simulink model "yangguo_Hermite_ISCAS2014_v03Final"  (Simulink 8.0)
settings: Solver=ode45  StartTime=0  StopTime=2e-8  FixedStep=Auto  MaxStep=1e-11  RelTol=1e-3
undefined symbols (not defined in the file or in its folder): tau
libraries: simulink x1
settings Model: Creator=yangguo  LastModifiedBy=Kushal
settings DataIOCC: SignalLoggingSaveFormat=ModelDataLogs
settings DebuggingCC: FcnCallInpInsideContextMsg=UseLocalSettings
settings GRTTargetCC: CombineOutputUpdateFcns=off  GRTInterface=on

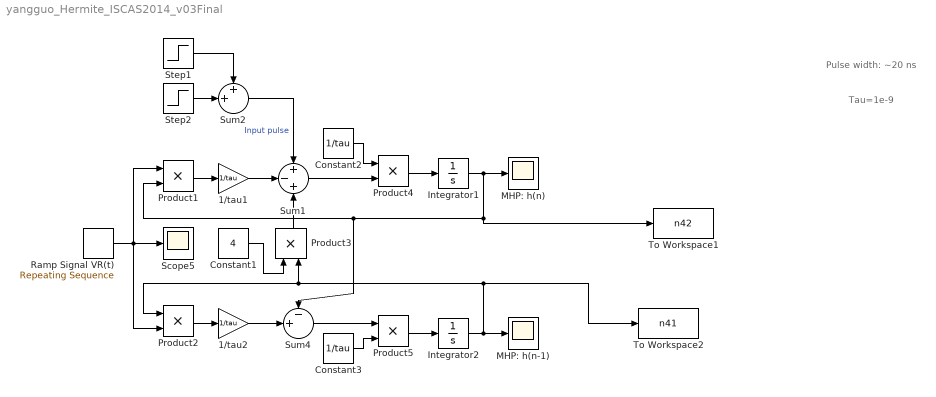
== system yangguo_Hermite_ISCAS2014_v03Final ==
  note: Tau=1e-9
  note: Pulse width: ~20 ns
  1/tau1 : Gain  Gain=1/tau
  1/tau2 : Gain  Gain=1/tau
  Constant1 : Constant  Value=4
  Constant2 : Constant  Value=1/tau
  Constant3 : Constant  Value=1/tau
  Integrator1 : Integrator
  Integrator2 : Integrator
  MHP: h(n) : Scope
      settings: TimeRange=1e-009  YMin=-10000000000000  YMax=10000000000000  SaveName=Hn1  MaxDataPoints=10000
  MHP: h(n-1) : Scope
      settings: SaveName=MHn1  MaxDataPoints=10000
  Product{1..5} (5 alike) : Product  RndMeth=Zero
  Ramp Signal VR(t) : simulink/Sources/Repeating Sequence  rep_seq_t=[0 20e-9]  rep_seq_y=[-5e-9 5e-9]
  Scope5 : Scope
      settings: TimeRange=1e-009  YMin=-10000000000000  YMax=10000000000000  SaveName=Output5  MaxDataPoints=10000
  Step1 : Step  Time=0.19e-8  After=-1e-3  SampleTime=0
  Step2 : Step  Time=0.2e-8  After=1e-3  SampleTime=0
  Sum1 : Sum  Inputs=+-+
  Sum2 : Sum  Inputs=++|
  Sum4 : Sum  Inputs=-+|
  To Workspace1 : ToWorkspace  VariableName=n42  SampleTime=-1
  To Workspace2 : ToWorkspace  VariableName=n41  SampleTime=-1
  wires:
  Constant1/1 -> Product3/1
  Product5/1 -> Integrator2/1
  Constant3/1 -> Product5/2
  Sum4/1 -> Product5/1
  Sum1/1 -> Product4/2
  Constant2/1 -> Product4/1
  Integrator2/1 -> Product2/1, Product3/2, To Workspace2/1, MHP: h(n-1)/1
  Step2/1 -> Sum2/2
  Step1/1 -> Sum2/1
  Sum2/1 -> Sum1/1  "Input pulse"
  Product4/1 -> Integrator1/1
  Product1/1 -> 1/tau1/1
  1/tau2/1 -> Sum4/2
  Product2/1 -> 1/tau2/1
  1/tau1/1 -> Sum1/2
  Product3/1 -> Sum1/3
  Ramp Signal VR(t)/1 -> Scope5/1, Product1/1, Product2/2
  Integrator1/1 -> To Workspace1/1, Sum4/1, Product1/2, MHP: h(n)/1
